simulink model "S_B_Custom_Model_2020a"  (R2020a)
settings: Solver=ode23t  StartTime=0.0  StopTime=6*3600  MaxStep=0.03  RelTol=1e-6
model workspace (MAT data in the model file):
  CHGTime55C = [12335 12235.3030303 12110.6060606 11985.9090909 11861.2121212 11737.2727273 11626.8181818 11502.1212121 11377.4242424 11252.7272727 11128.030303 11003.3333333 ... (100 elements, 100x1)]
  CHG_time25C = [14633.3333333 14511.9191919 14363.8383838 14215.7575758 14084.8484848 13949.5959596 13801.5151515 13653.4343434 13505.3535354 13357.2727273 13209.1919192 13061.1111111 ... (100 elements, 100x1)]
  CHG_time40C = [16740 16581.010101 16412.020202 16243.030303 16084.040404 15915.0505051 15746.0606061 15577.0707071 15408.0808081 15239.0909091 15070.1010101 14901.1111111 ... (100 elements, 100x1)]
  Capacity05A = [-5.0715 -5.02064646465 -4.96968686869 -4.91803030303 -4.86737373737 -4.81571717172 -4.76506060606 -4.7134040404 -4.6625 -4.61109090909 -4.55946969697 -4.50877777778 ... (100 elements, 100x1)]
  Capacity10A = [-4.9645 -4.91586363636 -4.86572727273 -4.81559090909 -4.76545454545 -4.71531818182 -4.66518181818 -4.61501515152 -4.5648030303 -4.51477272727 -4.46463636364 -4.4145 ... (100 elements, 100x1)]
  Capacity15A = [-4.9185 -4.87028282828 -4.82056565657 -4.77084848485 -4.72113131313 -4.67141414141 -4.6216969697 -4.57197979798 -4.52226262626 -4.47254545455 -4.42282828283 -4.37316666667 ... (100 elements, 100x1)]
  Capacity5A = [-4.989 -4.93917171717 -4.88857575758 -4.83801515152 -4.78815151515 -4.73743939394 -4.68672727273 -4.63701515152 -4.5863030303 -4.53559090909 -4.48566161616 -4.43516666667 ... (100 elements, 100x1)]
  Current05A = [0 0 0 0 0 0 0 0 0 0 0 0 ... (100 elements, 100x1)]
  Current10A = [-9.992 -9.9915 -9.9915 -9.9915 -9.9915 -9.9915 -9.9915 -9.9915 -9.9915 -9.9915 -9.9915 -9.9915 ... (100 elements, 100x1)]
  Current15A = [-14.99 -14.99 -14.99 -14.99 -14.99 -14.99 -14.99 -14.99 -14.99 -14.99 -14.99 -14.99 ... (100 elements, 100x1)]
  Current5A = [-4.9895 -4.99 -4.99 -4.99 -4.99 -4.99 -4.99 -4.99 -4.99 -4.99 -4.99 -4.99 ... (100 elements, 100x1)]
  DCHGCapacity55C = [-5.144 -5.09218686869 -5.04086363636 -4.98854545455 -4.93674747475 -4.88490909091 -4.83296969697 -4.78077272727 -4.72895454545 -4.67713636364 -4.62481818182 -4.57344444444 ... (100 elements, 100x1)]
  DCHGVoltage55C = [2.4995 2.64063636364 2.74113636364 2.81595454545 2.87527272727 2.92509090909 2.96940909091 3.00919191919 3.04500505051 3.07654545455 3.10455050505 3.1305 ... (100 elements, 100x1)]
  DCHG_capacity25C = [-5.128 -5.07663299663 -5.02509090909 -4.9733030303 -4.92151515152 -4.86972727273 -4.81780808081 -4.76607407407 -4.71405723906 -4.66254545455 -4.61078787879 -4.5587037037 ... (100 elements, 100x1)]
  DCHG_capacity40C = [-5.12166666667 -5.06995959596 -5.01858585859 -4.96687878788 -4.91483838384 -4.86309427609 -4.81175757576 -4.75971717172 -4.70812457912 -4.65663636364 -4.6045959596 -4.55281481481 ... (100 elements, 100x1)]
  DCHG_voltage25C = [2.5 2.64115824916 2.73824242424 2.81103030303 2.86915151515 2.91918518519 2.96385858586 3.00459259259 3.04133333333 3.07375757576 3.10317845118 3.13 ... (100 elements, 100x1)]
  DCHG_voltage40C = [2.5 2.64113804714 2.74026599327 2.81378787879 2.8727037037 2.92262962963 2.96757575758 3.00806734007 3.04432323232 3.07633333333 3.10490572391 3.1317037037 ... (100 elements, 100x1)]
  Param : Simulink.Parameter (value not decoded)
  RT05A = [0 0 0 0 0 0 0 0 0 0 0 0 ... (100 elements, 100x1)]
  RT10A = [0.000100080064051 0.00676736842478 0.0104184516435 0.0126167848732 0.0140700403424 0.015453539549 0.0166596152184 0.0175790836352 0.0182392407284 0.0185930768426 0.0188089168723 0.0189049581033 ... (100 elements, 100x1)]
  RT15A = [0 0.00554342625724 0.00881159830459 0.0109001960903 0.0124254553541 0.0137751767171 0.0148543473427 0.0157162013733 0.0163081785163 0.0167626902784 0.0170746827852 0.0171670002224 ... (100 elements, 100x1)]
  RT5A = [0.000100210441928 0.00482986174369 0.00833586364648 0.0106880427522 0.0123874010648 0.0139723892229 0.0155006983664 0.0166929819234 0.0176008582822 0.0181362725451 0.0185441590251 0.0187820084614 ... (100 elements, 100x1)]
  SOC05A = [0 0.0100273164455 0.0200755459555 0.0302612041742 0.0402496820716 0.0504353402904 0.0604238181878 0.0706094764066 0.0806467514542 0.0907836125227 0.10096229972 0.110957748639 ... (100 elements, 100x1)]
  SOC10A = [0 0.00979683022185 0.0198958056748 0.0299947811278 0.0400937565808 0.0501927320338 0.0602917074868 0.0703967868838 0.080511022197 0.0905886338458 0.100687609299 0.110786584752 ... (100 elements, 100x1)]
  SOC15A = [0 0.0098032269426 0.0199114249129 0.0300196228833 0.0401278208537 0.050236018824 0.0603442167944 0.0704524147647 0.0805606127351 0.0906688107054 0.100777008676 0.110873911423 ... (100 elements, 100x1)]
  SOC25C = [0 0.0100169663352 0.0200680754503 0.0301671157755 0.0402661561008 0.050365196426 0.0604898438362 0.0705783786907 0.0807220672665 0.0907672670543 0.100860398052 0.111017218467 ... (100 elements, 100x1)]
  SOC40C = [0 0.0100957508702 0.0201264187597 0.0302221696299 0.040383003481 0.0504859857935 0.0605094222406 0.0706702560917 0.0807436552311 0.0907966748513 0.100957508702 0.111067722457 ... (100 elements, 100x1)]
  SOC55C = [0 0.0100725371915 0.0200498374099 0.0302205570479 0.040290148766 0.0503675950799 0.060464677883 0.0706118337339 0.0806853527499 0.0907588717659 0.100929591404 0.110916709867 ... (100 elements, 100x1)]
  SOC5A = [0 0.00998762935023 0.0201291325765 0.0302635495059 0.040258265153 0.0504230519264 0.0605878386997 0.0705521845029 0.0807169712762 0.0908817580495 0.100889633962 0.111010890626 ... (100 elements, 100x1)]
  Voltage05A = [2.5 2.64131313131 2.73952020202 2.81396969697 2.87462626263 2.92878282828 2.97631818182 3.0185959596 3.05482828283 3.0865 3.11503535354 3.14022222222 ... (100 elements, 100x1)]
  Voltage10A = [2.499 2.5736969697 2.63542424242 2.68790909091 2.73404545455 2.77437878788 2.80986363636 2.84295454545 2.87259090909 2.90072727273 2.92710606061 2.95133333333 ... (100 elements, 100x1)]
  Voltage15A = [2.5 2.55821717172 2.60743434343 2.65057575758 2.68836868687 2.72229292929 2.75365151515 2.78301010101 2.81036868687 2.83522727273 2.85908585859 2.88288888889 ... (100 elements, 100x1)]
  Voltage5A = [2.4995 2.61721212121 2.69792424242 2.76063636364 2.81281313131 2.85906060606 2.89896969697 2.9352979798 2.967 2.996 3.0225 3.0465 ... (100 elements, 100x1)]
  temp25C = [302.063611111 302.097992144 302.124801908 302.108875421 302.09875982 302.038860831 301.993885522 302.043447811 301.958380471 302.027050505 302.022184063 301.955135802 ... (100 elements, 100x1)]
  temp40C = [311.240833333 312.174193603 312.448372054 312.47840404 312.481924242 312.475368687 312.536590909 312.636055556 312.60019697 312.601717172 312.619693603 312.584314815 ... (100 elements, 100x1)]
  temp55C = [327.716599383 327.643714956 327.735823245 327.782294302 327.755474781 327.740584002 327.757436513 327.776213951 327.720010617 327.727628249 327.697848259 327.730854322 ... (100 elements, 100x1)]
libraries: BatteryEstimators x1
(part 2 of 2)

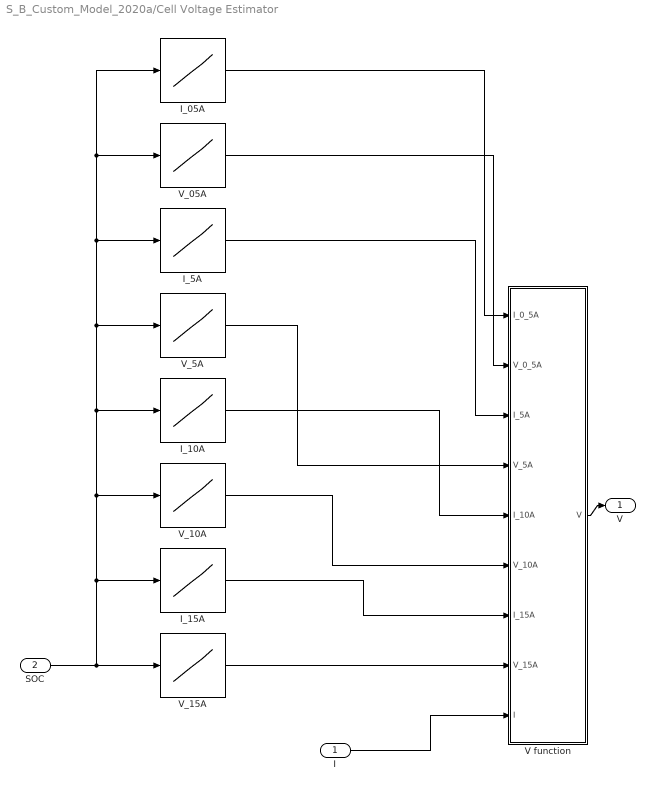
== system S_B_Custom_Model_2020a/Cell Voltage Estimator ==
  I : Inport
  SOC : Inport  Port=2
  I_05A : Lookup_n-D  NumberOfTableDimensions=1  BreakpointsForDimension1=SOC05A  Table=Current05A  InternalRulePriority=Speed  RndMeth=Simplest  InputSameDT=on
  I_10A : Lookup_n-D  NumberOfTableDimensions=1  BreakpointsForDimension1=SOC10A  Table=Current10A  InternalRulePriority=Speed  RndMeth=Simplest  InputSameDT=on
  I_15A : Lookup_n-D  NumberOfTableDimensions=1  BreakpointsForDimension1=SOC15A  Table=Current15A  InternalRulePriority=Speed  RndMeth=Simplest  InputSameDT=on
  I_5A : Lookup_n-D  NumberOfTableDimensions=1  BreakpointsForDimension1=SOC5A  Table=Current5A  InternalRulePriority=Speed  RndMeth=Simplest  InputSameDT=on
  V function : MATLAB Function  TreatAsAtomicUnit=on
  V_05A : Lookup_n-D  NumberOfTableDimensions=1  BreakpointsForDimension1=SOC05A  Table=Voltage05A  InternalRulePriority=Speed  RndMeth=Simplest  InputSameDT=on
  V_10A : Lookup_n-D  NumberOfTableDimensions=1  BreakpointsForDimension1=SOC10A  Table=Voltage10A  InternalRulePriority=Speed  RndMeth=Simplest  InputSameDT=on
  V_15A : Lookup_n-D  NumberOfTableDimensions=1  BreakpointsForDimension1=SOC15A  Table=Voltage15A  InternalRulePriority=Speed  RndMeth=Simplest  InputSameDT=on
  V_5A : Lookup_n-D  NumberOfTableDimensions=1  BreakpointsForDimension1=SOC5A  Table=Voltage5A  InternalRulePriority=Speed  RndMeth=Simplest  InputSameDT=on
  V : Outport
  wires:
  V function/1(V) -> V/1
  I/1 -> V function/9(I)
  V_15A/1 -> V function/8(V_15A)
  I_15A/1 -> V function/7(I_15A)
  V_10A/1 -> V function/6(V_10A)
  I_10A/1 -> V function/5(I_10A)
  V_5A/1 -> V function/4(V_5A)
  I_5A/1 -> V function/3(I_5A)
  V_05A/1 -> V function/2(V_0_5A)
  I_05A/1 -> V function/1(I_0_5A)
  SOC/1 -> I_05A/1, V_05A/1, I_5A/1, V_5A/1, I_10A/1, V_10A/1, I_15A/1, V_15A/1

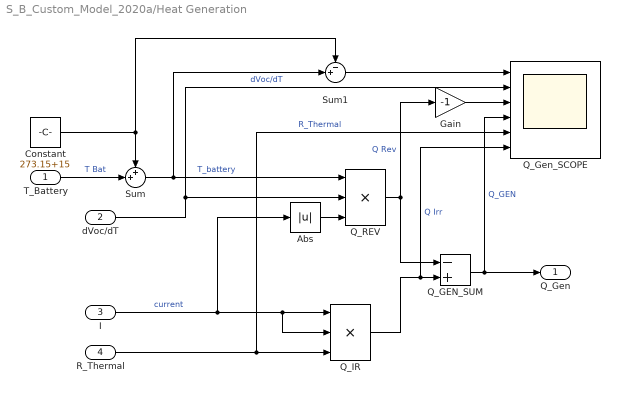
== system S_B_Custom_Model_2020a/Heat Generation ==
  T_Battery : Inport
  dVoc/dT : Inport  Port=2
  I : Inport  Port=3
  R_Thermal : Inport  Port=4
  Abs : Abs
  Constant : Constant  Value=273.15+15
  Gain : Gain  Gain=-1
  Q_GEN_SUM : Sum  Inputs=-+
  Q_Gen_SCOPE : Scope  NumInputPorts=6
  Q_IR : Product  Inputs=3
  Q_REV : Product  Inputs=3
  Sum : Sum  Inputs=++|
  Sum1 : Sum  Inputs=-+|
  Q_Gen : Outport
  wires:
  Q_REV/1 -> Q_GEN_SUM/1, Gain/1  "Q Rev"
  I/1 -> Q_IR/2, Q_IR/1, Abs/1  "current"
  R_Thermal/1 -> Q_IR/3, Q_Gen_SCOPE/5  "R_Thermal"
  Q_IR/1 -> Q_Gen_SCOPE/6, Q_GEN_SUM/2  "Q Irr"
  dVoc/dT/1 -> Q_REV/2, Q_Gen_SCOPE/2  "dVoc/dT"
  Q_GEN_SUM/1 -> Q_Gen_SCOPE/4, Q_Gen/1  "Q_GEN"
  Abs/1 -> Q_REV/3
  T_Battery/1 -> Sum/2  "T Bat"
  Constant/1 -> Sum1/1, Sum/1
  Sum/1 -> Sum1/2, Q_REV/1  "T_battery"
  Sum1/1 -> Q_Gen_SCOPE/1
  Gain/1 -> Q_Gen_SCOPE/3

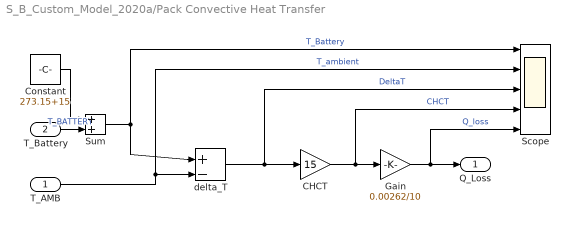
== system S_B_Custom_Model_2020a/Pack Convective Heat Transfer ==
  T_AMB : Inport
  T_Battery : Inport  Port=2
  CHCT : Gain  Gain=15
  Constant : Constant  Value=273.15+15
  Gain : Gain  Gain=0.00262/10
  Scope : Scope  NumInputPorts=5
  Sum : Sum  Inputs=+|+
  delta_T : Sum  Inputs=+|-
  Q_Loss : Outport
  wires:
  T_AMB/1 -> Scope/2, delta_T/2  "T_ambient"
  delta_T/1 -> Scope/3, CHCT/1  "DeltaT"
  CHCT/1 -> Scope/4, Gain/1  "CHCT"
  Gain/1 -> Scope/5, Q_Loss/1  "Q_loss"
  T_Battery/1 -> Sum/2  "T_BATTERY"
  Sum/1 -> delta_T/1, Scope/1  "T_Battery"
  Constant/1 -> Sum/1

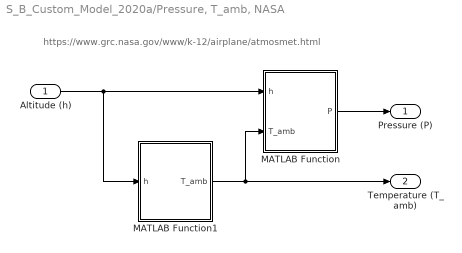
== system S_B_Custom_Model_2020a/Pressure, T_amb, NASA ==
  note: https://www.grc.nasa.gov/www/k-12/airplane/atmosmet.html
  Altitude (h) : Inport
  MATLAB Function : MATLAB Function  TreatAsAtomicUnit=on
  MATLAB Function1 : MATLAB Function  TreatAsAtomicUnit=on
  Pressure (P) : Outport
  Temperature (T_amb) : Outport  Port=2
  wires:
  MATLAB Function1/1(T_amb) -> MATLAB Function/2(T_amb), Temperature (T_amb)/1
  MATLAB Function/1(P) -> Pressure (P)/1
  Altitude (h)/1 -> MATLAB Function/1(h), MATLAB Function1/1(h)

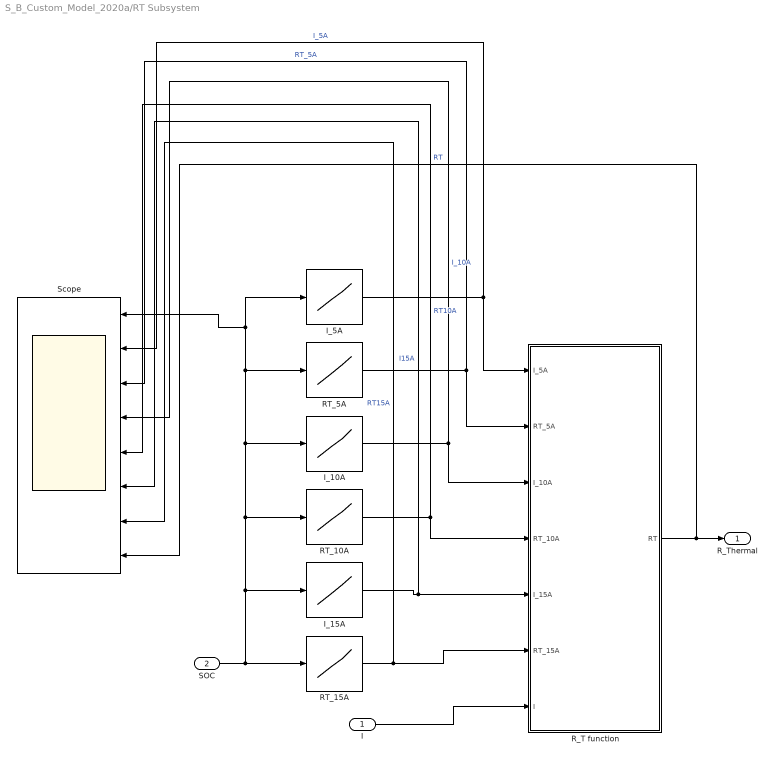
== system S_B_Custom_Model_2020a/RT Subsystem ==
  I : Inport
  SOC : Inport  Port=2
  I_10A : Lookup_n-D  NumberOfTableDimensions=1  BreakpointsForDimension1=SOC10A  Table=Current10A  InternalRulePriority=Speed  RndMeth=Simplest  InputSameDT=on
  I_15A : Lookup_n-D  NumberOfTableDimensions=1  BreakpointsForDimension1=SOC15A  Table=Current15A  InternalRulePriority=Speed  RndMeth=Simplest  InputSameDT=on
  I_5A : Lookup_n-D  NumberOfTableDimensions=1  BreakpointsForDimension1=SOC5A  Table=Current5A  InternalRulePriority=Speed  RndMeth=Simplest  InputSameDT=on
  RT_10A : Lookup_n-D  NumberOfTableDimensions=1  BreakpointsForDimension1=SOC10A  Table=RT10A  InternalRulePriority=Speed  RndMeth=Simplest  InputSameDT=on
  RT_15A : Lookup_n-D  NumberOfTableDimensions=1  BreakpointsForDimension1=SOC15A  Table=RT15A  InternalRulePriority=Speed  RndMeth=Simplest  InputSameDT=on
  RT_5A : Lookup_n-D  NumberOfTableDimensions=1  BreakpointsForDimension1=SOC5A  Table=RT5A  InternalRulePriority=Speed  RndMeth=Simplest  InputSameDT=on
  R_T function : MATLAB Function  TreatAsAtomicUnit=on
  Scope : Scope  NumInputPorts=8
  R_Thermal : Outport
  wires:
  R_T function/1(RT) -> Scope/8, R_Thermal/1  "RT"
  I/1 -> R_T function/7(I)
  SOC/1 -> RT_5A/1, I_5A/1, Scope/1, I_10A/1, RT_10A/1, I_15A/1, RT_15A/1
  I_5A/1 -> R_T function/1(I_5A), Scope/2  "I_5A"
  RT_5A/1 -> R_T function/2(RT_5A), Scope/3  "RT_5A"
  I_10A/1 -> R_T function/3(I_10A), Scope/4  "I_10A"
  RT_10A/1 -> R_T function/4(RT_10A), Scope/5  "RT10A"
  I_15A/1 -> Scope/6, R_T function/5(I_15A)  "I15A"
  RT_15A/1 -> Scope/7, R_T function/6(RT_15A)  "RT15A"

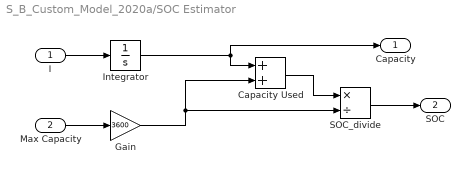
== system S_B_Custom_Model_2020a/SOC Estimator ==
  I : Inport
  Max Capacity : Inport  Port=2
  Capacity Used : Sum
  Gain : Gain  Gain=3600
  Integrator : Integrator
  SOC_divide : Product  Inputs=*/
  Capacity : Outport
  SOC : Outport  Port=2
  wires:
  Capacity Used/1 -> SOC_divide/1
  SOC_divide/1 -> SOC/1
  I/1 -> Integrator/1
  Max Capacity/1 -> Gain/1
  Gain/1 -> SOC_divide/2, Capacity Used/2
  Integrator/1 -> Capacity Used/1, Capacity/1

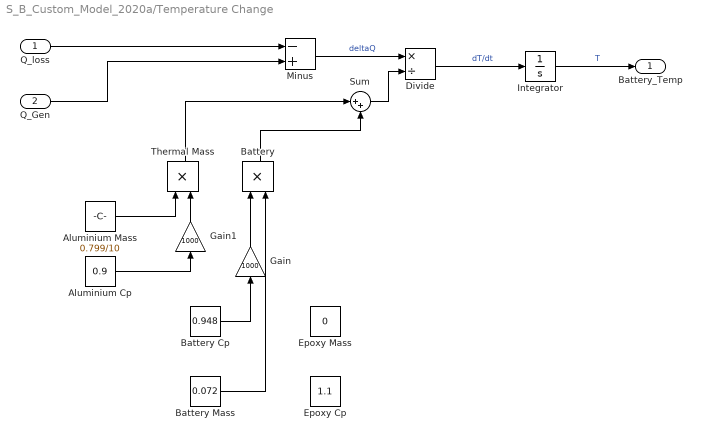
== system S_B_Custom_Model_2020a/Temperature Change ==
  Q_loss : Inport
  Q_Gen : Inport  Port=2
  Aluminium Cp : Constant  Value=0.9  VectorParams1D=off
  Aluminium Mass : Constant  Value=0.799/10  VectorParams1D=off
  Battery : Product  OutDataTypeStr=double
  Battery Cp : Constant  Value=0.948  VectorParams1D=off
  Battery Mass : Constant  Value=0.072  VectorParams1D=off
  Divide : Product  Inputs=*/
  Epoxy Cp : Constant  Value=1.1  VectorParams1D=off
  Epoxy Mass : Constant  Value=0  VectorParams1D=off
  Gain : Gain  Gain=1000
  Gain1 : Gain  Gain=1000
  Integrator : Integrator
  Minus : Sum  Inputs=-+
  Sum : Sum  Inputs=|++
  Thermal Mass : Product  OutDataTypeStr=double
  Battery_Temp : Outport
  wires:
  Integrator/1 -> Battery_Temp/1  "T"
  Battery/1 -> Sum/2
  Divide/1 -> Integrator/1  "dT/dt"
  Minus/1 -> Divide/1  "deltaQ"
  Sum/1 -> Divide/2
  Battery Cp/1 -> Gain/1
  Aluminium Cp/1 -> Gain1/1
  Aluminium Mass/1 -> Thermal Mass/1
  Q_loss/1 -> Minus/1
  Q_Gen/1 -> Minus/2
  Battery Mass/1 -> Battery/2
  Gain/1 -> Battery/1
  Thermal Mass/1 -> Sum/1
  Gain1/1 -> Thermal Mass/2

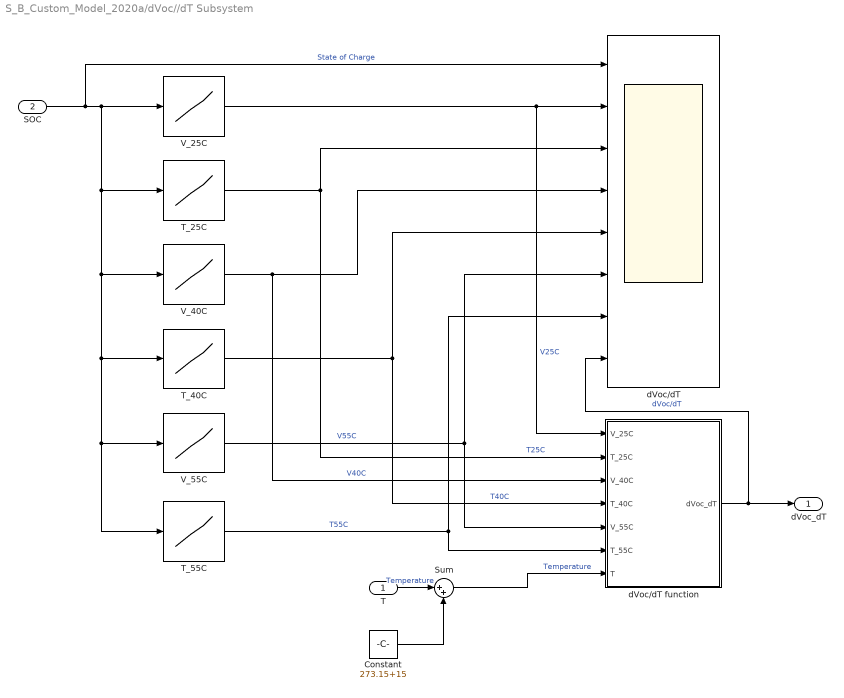
== system S_B_Custom_Model_2020a/dVoc//dT Subsystem ==
  T : Inport
  SOC : Inport  Port=2
  Constant : Constant  Value=273.15+15
  Sum : Sum  Inputs=|++
  T_25C : Lookup_n-D  NumberOfTableDimensions=1  BreakpointsForDimension1=SOC25C  Table=temp25C  InternalRulePriority=Speed  RndMeth=Simplest  InputSameDT=on
  T_40C : Lookup_n-D  NumberOfTableDimensions=1  BreakpointsForDimension1=SOC40C  Table=temp40C  InternalRulePriority=Speed  RndMeth=Simplest  InputSameDT=on
  T_55C : Lookup_n-D  NumberOfTableDimensions=1  BreakpointsForDimension1=SOC55C  Table=temp55C  InternalRulePriority=Speed  RndMeth=Simplest  InputSameDT=on
  V_25C : Lookup_n-D  NumberOfTableDimensions=1  BreakpointsForDimension1=SOC25C  Table=DCHG_voltage25C  InternalRulePriority=Speed  RndMeth=Simplest  InputSameDT=on
  V_40C : Lookup_n-D  NumberOfTableDimensions=1  BreakpointsForDimension1=SOC40C  Table=DCHG_voltage40C  InternalRulePriority=Speed  RndMeth=Simplest  InputSameDT=on
  V_55C : Lookup_n-D  NumberOfTableDimensions=1  BreakpointsForDimension1=SOC55C  Table=DCHGVoltage55C  InternalRulePriority=Speed  RndMeth=Simplest  InputSameDT=on
  dVoc/dT : Scope  NumInputPorts=8
  dVoc/dT function : MATLAB Function  TreatAsAtomicUnit=on
  dVoc_dT : Outport
  wires:
  Sum/1 -> dVoc/dT function/7(T)  "Temperature"
  dVoc/dT function/1(dVoc_dT) -> dVoc/dT/8, dVoc_dT/1  "dVoc/dT"
  V_25C/1 -> dVoc/dT function/1(V_25C), dVoc/dT/2  "V25C"
  T_25C/1 -> dVoc/dT function/2(T_25C), dVoc/dT/3  "T25C"
  V_40C/1 -> dVoc/dT function/3(V_40C), dVoc/dT/4  "V40C"
  T_40C/1 -> dVoc/dT function/4(T_40C), dVoc/dT/5  "T40C"
  V_55C/1 -> dVoc/dT function/5(V_55C), dVoc/dT/6  "V55C"
  T_55C/1 -> dVoc/dT/7, dVoc/dT function/6(T_55C)  "T55C"
  SOC/1 -> dVoc/dT/1, T_55C/1, V_55C/1, T_40C/1, V_40C/1, T_25C/1, V_25C/1  "State of Charge"
  T/1 -> Sum/1  "Temperature"
  Constant/1 -> Sum/2

== matlab function S_B_Custom_Model_2020a/RT Subsystem/R_T function ==
  data: I_5A input; RT_5A input; I_10A input; RT output; RT_10A input; I_15A input; RT_15A input; I input
function RT = fcn(I_5A,RT_5A, I_10A,RT_10A, I_15A,RT_15A, I)
    
    %Current Index
    a= I_5A;
    b= I_10A;
    c= I_15A;

    %Lagrange polynomial 
  
    Rt_1C = RT_5A .* (I-b) .* (I-c)  ./ ((a-b) .* (a-c) ); 
    Rt_2C = RT_10A .* (I-a) .* (I-c) ./ ((b-a) .* (b-c) );
    Rt_3C = RT_15A .* (I-a) .* (I-b) ./ ((c-a) .* (c-b) );

    RT = Rt_1C + Rt_2C + Rt_3C; 

end

== matlab function S_B_Custom_Model_2020a/dVoc//dT Subsystem/dVoc//dT function ==
  data: V_25C input; T_25C input; V_40C input; T_40C input; V_55C input; T_55C input; T input; dVoc_dT output
function dVoc_dT = fcn(V_25C,T_25C, V_40C,T_40C, V_55C,T_55C,  T)

    dVoc_25C = V_25C .* (2*T - T_40C - T_55C) / ( (T_25C - T_40C ) * (T_25C - T_55C) ); 
    dVoc_40C = V_40C .* (2*T - T_25C - T_55C) / ( (T_40C - T_25C ) * (T_40C - T_55C ) ); 
    dVoc_55C = V_55C .* (2*T - T_25C - T_40C) / ( (T_55C - T_25C ) * (T_55C - T_40C ) );

    %Output
    dVoc_dT = double(dVoc_25C + dVoc_40C + dVoc_55C); 
    
end

== matlab function S_B_Custom_Model_2020a/Cell Voltage Estimator/V function ==
  data: I_0_5A input; V_0_5A input; I_5A input; V_5A input; I_10A input; V output; V_10A input; I_15A input; V_15A input; I input
function V = fcn(I_0_5A,V_0_5A, I_5A,V_5A, I_10A,V_10A, I_15A,V_15A, I)
    

    a= I_0_5A;
    b= I_5A;
    c= I_10A;
    d= I_15A;

    %Lagrange polynomial 
    Rt_0_1C = V_0_5A .* (I-b) .*(I-c) .* (I-d) ./ ((a-b) .* (a-c) .* (a-d) );
    Rt_1C = V_5A .* (I-a) .* (I-c) .* (I-d) ./ ((b-a) .* (b-c) .* (b-d) ); 
    Rt_2C = V_10A .* (I-a) .* (I-b) .* (I-d) ./ ((c-a) .* (c-b) .* (c-d) );
    Rt_3C = V_15A .* (I-a) .* (I-b) .* (I-c) ./ ((d-a) .* (d-b) .* (d-c) );

    V = double( Rt_0_1C + Rt_1C + Rt_2C + Rt_3C ); 

end

== matlab function S_B_Custom_Model_2020a/Pressure, T_amb, NASA/MATLAB Function ==
  data: h input; P output; T_amb input
function P = Pressure(h, T_amb)
    if h>=25000
        P = 2.488 * (T_amb/216.6).^(-11.388) *10^3 ;%Pressure, kPa
    elseif (h >= 11000) && (h<=25000)
        P = 22.65*exp(1.73-0.000157*h) ;%Pressure, kPa
    elseif h>= 11000 
        P =101.29*(T_amb/288.08).^(5.256) ;%Pressure, kPa 
    else 
        P=0;
    end
end

== matlab function S_B_Custom_Model_2020a/Pressure, T_amb, NASA/MATLAB Function1 ==
  data: h input; T_amb output
function T_amb = Temperature(h)
    if h>=25000
        T_amb =-131.21+0.00299*h + 273.15 ;%T_amb, kelvin
    elseif (h >= 11000) && (h<=25000)
        T_amb = -56.46 +273.15; %T_amb, kelvin
    elseif h>= 11000 
        T_amb = 15.04-0.00649*h + 273.15; %T_amb, kelvin 
    else 
        T_amb = 0;
    end
end
